simulink model "REL"  (R2022a)
settings: Solver=FixedStepDiscrete  StartTime=0.0  StopTime=10.0  FixedStep=0.01  RelTol=1e-3
libraries: simulink x8, DoorRatSts x4, DoorRlsDriver x2, DoorRlsReq x2
settings Model: Creator=DELL  LastModifiedBy=DELL
settings DataIOCC: SaveFormat=StructureWithTime
settings OptimizationCC: DefaultParameterBehavior=Inlined  EnhancedBackFolding=on  PassReuseOutputArgsAs=Individual arguments  ZeroExternalMemoryAtStartup=off  ZeroInternalMemoryAtStartup=off  OptimizeBlockOrder=speed  DifferentSizesBufferReuse=on  OptimizationCustomize=off  EfficientTunableParamExpr=on
settings DebuggingCC: ParameterTunabilityLossMsg=error
settings ModelReferenceCC: ModelReferenceNumInstancesAllowed=Single
settings SFSimCC: MATLABDynamicMemAlloc=off
settings RTWCC: Description=AUTOSAR  SystemTargetFile=autosar.tlc  GenCodeOnly=on  TemplateMakefile=ert_default_tmf
settings CodeAppCC: ForceParamTrailComments=on  IgnoreCustomStorageClasses=off  OperatorAnnotations=on  SimulinkDataObjDesc=on  SFDataObjDesc=on  InsertBlockDesc=on
settings STFCustomTargetCC: TargetLangStandard=C99 (ISO)  MultiwordLength=256  ParMdlRefBuildCompliant=on  CompOptLevelCompliant=on  IncludeMdlTerminateFcn=off  CombineOutputUpdateFcns=on  SuppressErrorStatus=on  ERTCustomFileBanners=on  SupportNonFinite=off  SupportComplex=off  SupportContinuousTime=off  SupportNonInlinedSFcns=off  RemoveResetFunc=on  MATLABClassNameForMDSCustomization=Simulink.SoftwareTarget.ERTCustomization  AutosarCompliant=on  GRTInterface=off  UseToolchainInfoCompliant=on  LookupTableObjectStructAxisOrder=2,1,3,4,...  LUTObjectStructOrderEvenSpacing=Size,Table,Breakpoints  SystemTargetFile=autosar.tlc
settings ERTTargetCC: TargetLangStandard=C99 (ISO)  ConcurrentExecutionCompliant=off  IncludeMdlTerminateFcn=off  SuppressErrorStatus=on  SupportNonFinite=off  SupportComplex=off  ModelStepFunctionPrototypeControlCompliant=off  CPPClassGenCompliant=off  AutosarCompliant=on  LookupTableObjectStructAxisOrder=2,1,3,4,...  LUTObjectStructOrderEvenSpacing=Size,Table,Breakpoints  InlinedParameterPlacement=NonHierarchical  ERTCustomFileTemplate=example_file_process.tlc

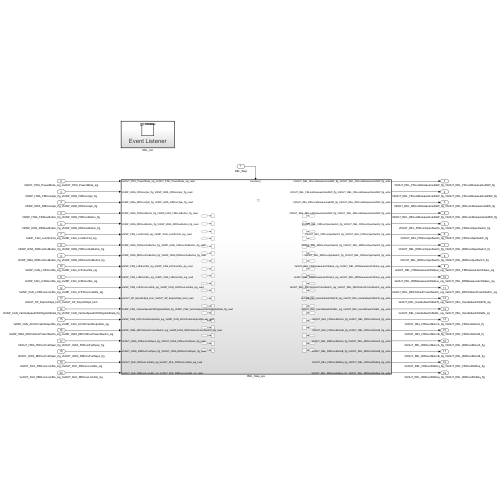
[thumbnail: Simulink's stored preview of the top-level diagram]
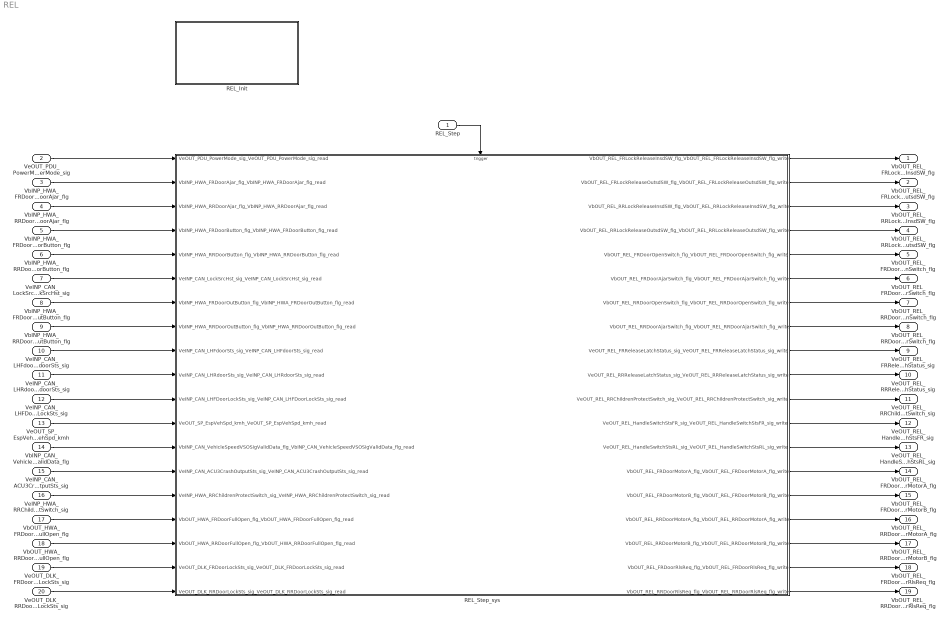
== system REL ==
  REL_Step : Inport  SampleTime=0.01  OutputFunctionCall=on
  VeOUT_PDU_PowerMode_sig_VeOUT_PDU_PowerMode_sig : Inport  Port=2  OutDataTypeStr=UInt8  PortDimensions=1
  VbINP_HWA_FRDoorAjar_flg_VbINP_HWA_FRDoorAjar_flg : Inport  Port=3  OutDataTypeStr=Boolean  PortDimensions=1
  VbINP_HWA_RRDoorAjar_flg_VbINP_HWA_RRDoorAjar_flg : Inport  Port=4  OutDataTypeStr=Boolean  PortDimensions=1
  VbINP_HWA_FRDoorButton_flg_VbINP_HWA_FRDoorButton_flg : Inport  Port=5  OutDataTypeStr=Boolean  PortDimensions=1
  VbINP_HWA_RRDoorButton_flg_VbINP_HWA_RRDoorButton_flg : Inport  Port=6  OutDataTypeStr=Boolean  PortDimensions=1
  VeINP_CAN_LockSrcHst_sig_VeINP_CAN_LockSrcHst_sig : Inport  Port=7  OutDataTypeStr=UInt8  PortDimensions=1
  VbINP_HWA_FRDoorOutButton_flg_VbINP_HWA_FRDoorOutButton_flg : Inport  Port=8  OutDataTypeStr=Boolean  PortDimensions=1
  VbINP_HWA_RRDoorOutButton_flg_VbINP_HWA_RRDoorOutButton_flg : Inport  Port=9  OutDataTypeStr=Boolean  PortDimensions=1
  VeINP_CAN_LHFdoorSts_sig_VeINP_CAN_LHFdoorSts_sig : Inport  Port=10  OutDataTypeStr=UInt8  PortDimensions=1
  VeINP_CAN_LHRdoorSts_sig_VeINP_CAN_LHRdoorSts_sig : Inport  Port=11  OutDataTypeStr=UInt8  PortDimensions=1
  VeINP_CAN_LHFDoorLockSts_sig_VeINP_CAN_LHFDoorLockSts_sig : Inport  Port=12  OutDataTypeStr=UInt8  PortDimensions=1
  VeOUT_SP_EspVehSpd_kmh_VeOUT_SP_EspVehSpd_kmh : Inport  Port=13  OutDataTypeStr=UInt8  PortDimensions=1
  VbINP_CAN_VehicleSpeedVSOSigValidData_flg_VbINP_CAN_VehicleSpeedVSOSigValidData_flg : Inport  Port=14  OutDataTypeStr=Boolean  PortDimensions=1
  VeINP_CAN_ACU3CrashOutputSts_sig_VeINP_CAN_ACU3CrashOutputSts_sig : Inport  Port=15  OutDataTypeStr=UInt8  PortDimensions=1
  VeINP_HWA_RRChildrenProtectSwitch_sig_VeINP_HWA_RRChildrenProtectSwitch_sig : Inport  Port=16  OutDataTypeStr=UInt8  PortDimensions=1
  VbOUT_HWA_FRDoorFullOpen_flg_VbOUT_HWA_FRDoorFullOpen_flg : Inport  Port=17  OutDataTypeStr=Boolean  PortDimensions=1
  VbOUT_HWA_RRDoorFullOpen_flg_VbOUT_HWA_RRDoorFullOpen_flg : Inport  Port=18  OutDataTypeStr=Boolean  PortDimensions=1
  VeOUT_DLK_FRDoorLockSts_sig_VeOUT_DLK_FRDoorLockSts_sig : Inport  Port=19  OutDataTypeStr=UInt8  PortDimensions=1
  VeOUT_DLK_RRDoorLockSts_sig_VeOUT_DLK_RRDoorLockSts_sig : Inport  Port=20  OutDataTypeStr=UInt8  PortDimensions=1
  REL_Init : Subsystem
  REL_Step_sys : Subsystem
  VbOUT_REL_FRLockReleaseInsdSW_flg_VbOUT_REL_FRLockReleaseInsdSW_flg : Outport  OutDataTypeStr=Boolean  PortDimensions=1
  VbOUT_REL_FRLockReleaseOutsdSW_flg_VbOUT_REL_FRLockReleaseOutsdSW_flg : Outport  Port=2  OutDataTypeStr=Boolean  PortDimensions=1
  VbOUT_REL_RRLockReleaseInsdSW_flg_VbOUT_REL_RRLockReleaseInsdSW_flg : Outport  Port=3  OutDataTypeStr=Boolean  PortDimensions=1
  VbOUT_REL_RRLockReleaseOutsdSW_flg_VbOUT_REL_RRLockReleaseOutsdSW_flg : Outport  Port=4  OutDataTypeStr=Boolean  PortDimensions=1
  VbOUT_REL_FRDoorOpenSwitch_flg_VbOUT_REL_FRDoorOpenSwitch_flg : Outport  Port=5  OutDataTypeStr=Boolean  PortDimensions=1
  VbOUT_REL_FRDoorAjarSwitch_flg_VbOUT_REL_FRDoorAjarSwitch_flg : Outport  Port=6  OutDataTypeStr=Boolean  PortDimensions=1
  VbOUT_REL_RRDoorOpenSwitch_flg_VbOUT_REL_RRDoorOpenSwitch_flg : Outport  Port=7  OutDataTypeStr=Boolean  PortDimensions=1
  VbOUT_REL_RRDoorAjarSwitch_flg_VbOUT_REL_RRDoorAjarSwitch_flg : Outport  Port=8  OutDataTypeStr=Boolean  PortDimensions=1
  VeOUT_REL_FRReleaseLatchStatus_sig_VeOUT_REL_FRReleaseLatchStatus_sig : Outport  Port=9  OutDataTypeStr=UInt8  PortDimensions=1
  VeOUT_REL_RRReleaseLatchStatus_sig_VeOUT_REL_RRReleaseLatchStatus_sig : Outport  Port=10  OutDataTypeStr=UInt8  PortDimensions=1
  VeOUT_REL_RRChildrenProtectSwitch_sig_VeOUT_REL_RRChildrenProtectSwitch_sig : Outport  Port=11  OutDataTypeStr=UInt8  PortDimensions=1
  VeOUT_REL_HandleSwitchStsFR_sig_VeOUT_REL_HandleSwitchStsFR_sig : Outport  Port=12  OutDataTypeStr=UInt8  PortDimensions=1
  VeOUT_REL_HandleSwitchStsRL_sig_VeOUT_REL_HandleSwitchStsRL_sig : Outport  Port=13  OutDataTypeStr=UInt8  PortDimensions=1
  VbOUT_REL_FRDoorMotorA_flg_VbOUT_REL_FRDoorMotorA_flg : Outport  Port=14  OutDataTypeStr=Boolean  PortDimensions=1
  VbOUT_REL_FRDoorMotorB_flg_VbOUT_REL_FRDoorMotorB_flg : Outport  Port=15  OutDataTypeStr=Boolean  PortDimensions=1
  VbOUT_REL_RRDoorMotorA_flg_VbOUT_REL_RRDoorMotorA_flg : Outport  Port=16  OutDataTypeStr=Boolean  PortDimensions=1
  VbOUT_REL_RRDoorMotorB_flg_VbOUT_REL_RRDoorMotorB_flg : Outport  Port=17  OutDataTypeStr=Boolean  PortDimensions=1
  VbOUT_REL_FRDoorRlsReq_flg_VbOUT_REL_FRDoorRlsReq_flg : Outport  Port=18  OutDataTypeStr=Boolean  PortDimensions=1
  VbOUT_REL_RRDoorRlsReq_flg_VbOUT_REL_RRDoorRlsReq_flg : Outport  Port=19  OutDataTypeStr=Boolean  PortDimensions=1
  wires:
  VeOUT_PDU_PowerMode_sig_VeOUT_PDU_PowerMode_sig/1 -> REL_Step_sys/1(VeOUT_PDU_PowerMode_sig_VeOUT_PDU_PowerMode_sig_read)
  VbINP_HWA_FRDoorAjar_flg_VbINP_HWA_FRDoorAjar_flg/1 -> REL_Step_sys/2(VbINP_HWA_FRDoorAjar_flg_VbINP_HWA_FRDoorAjar_flg_read)
  VbINP_HWA_RRDoorAjar_flg_VbINP_HWA_RRDoorAjar_flg/1 -> REL_Step_sys/3(VbINP_HWA_RRDoorAjar_flg_VbINP_HWA_RRDoorAjar_flg_read)
  VbINP_HWA_FRDoorButton_flg_VbINP_HWA_FRDoorButton_flg/1 -> REL_Step_sys/4(VbINP_HWA_FRDoorButton_flg_VbINP_HWA_FRDoorButton_flg_read)
  VbINP_HWA_RRDoorButton_flg_VbINP_HWA_RRDoorButton_flg/1 -> REL_Step_sys/5(VbINP_HWA_RRDoorButton_flg_VbINP_HWA_RRDoorButton_flg_read)
  VeINP_CAN_LockSrcHst_sig_VeINP_CAN_LockSrcHst_sig/1 -> REL_Step_sys/6(VeINP_CAN_LockSrcHst_sig_VeINP_CAN_LockSrcHst_sig_read)
  VbINP_HWA_FRDoorOutButton_flg_VbINP_HWA_FRDoorOutButton_flg/1 -> REL_Step_sys/7(VbINP_HWA_FRDoorOutButton_flg_VbINP_HWA_FRDoorOutButton_flg_read)
  VbINP_HWA_RRDoorOutButton_flg_VbINP_HWA_RRDoorOutButton_flg/1 -> REL_Step_sys/8(VbINP_HWA_RRDoorOutButton_flg_VbINP_HWA_RRDoorOutButton_flg_read)
  VeINP_CAN_LHFdoorSts_sig_VeINP_CAN_LHFdoorSts_sig/1 -> REL_Step_sys/9(VeINP_CAN_LHFdoorSts_sig_VeINP_CAN_LHFdoorSts_sig_read)
  VeINP_CAN_LHRdoorSts_sig_VeINP_CAN_LHRdoorSts_sig/1 -> REL_Step_sys/10(VeINP_CAN_LHRdoorSts_sig_VeINP_CAN_LHRdoorSts_sig_read)
  VeINP_CAN_LHFDoorLockSts_sig_VeINP_CAN_LHFDoorLockSts_sig/1 -> REL_Step_sys/11(VeINP_CAN_LHFDoorLockSts_sig_VeINP_CAN_LHFDoorLockSts_sig_read)
  VeOUT_SP_EspVehSpd_kmh_VeOUT_SP_EspVehSpd_kmh/1 -> REL_Step_sys/12(VeOUT_SP_EspVehSpd_kmh_VeOUT_SP_EspVehSpd_kmh_read)
  VbINP_CAN_VehicleSpeedVSOSigValidData_flg_VbINP_CAN_VehicleSpeedVSOSigValidData_flg/1 -> REL_Step_sys/13(VbINP_CAN_VehicleSpeedVSOSigValidData_flg_VbINP_CAN_VehicleSpeedVSOSigValidData_flg_read)
  VeINP_CAN_ACU3CrashOutputSts_sig_VeINP_CAN_ACU3CrashOutputSts_sig/1 -> REL_Step_sys/14(VeINP_CAN_ACU3CrashOutputSts_sig_VeINP_CAN_ACU3CrashOutputSts_sig_read)
  VeINP_HWA_RRChildrenProtectSwitch_sig_VeINP_HWA_RRChildrenProtectSwitch_sig/1 -> REL_Step_sys/15(VeINP_HWA_RRChildrenProtectSwitch_sig_VeINP_HWA_RRChildrenProtectSwitch_sig_read)
  VbOUT_HWA_FRDoorFullOpen_flg_VbOUT_HWA_FRDoorFullOpen_flg/1 -> REL_Step_sys/16(VbOUT_HWA_FRDoorFullOpen_flg_VbOUT_HWA_FRDoorFullOpen_flg_read)
  VbOUT_HWA_RRDoorFullOpen_flg_VbOUT_HWA_RRDoorFullOpen_flg/1 -> REL_Step_sys/17(VbOUT_HWA_RRDoorFullOpen_flg_VbOUT_HWA_RRDoorFullOpen_flg_read)
  VeOUT_DLK_FRDoorLockSts_sig_VeOUT_DLK_FRDoorLockSts_sig/1 -> REL_Step_sys/18(VeOUT_DLK_FRDoorLockSts_sig_VeOUT_DLK_FRDoorLockSts_sig_read)
  VeOUT_DLK_RRDoorLockSts_sig_VeOUT_DLK_RRDoorLockSts_sig/1 -> REL_Step_sys/19(VeOUT_DLK_RRDoorLockSts_sig_VeOUT_DLK_RRDoorLockSts_sig_read)
  REL_Step_sys/1(VbOUT_REL_FRLockReleaseInsdSW_flg_VbOUT_REL_FRLockReleaseInsdSW_flg_write) -> VbOUT_REL_FRLockReleaseInsdSW_flg_VbOUT_REL_FRLockReleaseInsdSW_flg/1
  REL_Step_sys/2(VbOUT_REL_FRLockReleaseOutsdSW_flg_VbOUT_REL_FRLockReleaseOutsdSW_flg_write) -> VbOUT_REL_FRLockReleaseOutsdSW_flg_VbOUT_REL_FRLockReleaseOutsdSW_flg/1
  REL_Step_sys/3(VbOUT_REL_RRLockReleaseInsdSW_flg_VbOUT_REL_RRLockReleaseInsdSW_flg_write) -> VbOUT_REL_RRLockReleaseInsdSW_flg_VbOUT_REL_RRLockReleaseInsdSW_flg/1
  REL_Step_sys/4(VbOUT_REL_RRLockReleaseOutsdSW_flg_VbOUT_REL_RRLockReleaseOutsdSW_flg_write) -> VbOUT_REL_RRLockReleaseOutsdSW_flg_VbOUT_REL_RRLockReleaseOutsdSW_flg/1
  REL_Step_sys/5(VbOUT_REL_FRDoorOpenSwitch_flg_VbOUT_REL_FRDoorOpenSwitch_flg_write) -> VbOUT_REL_FRDoorOpenSwitch_flg_VbOUT_REL_FRDoorOpenSwitch_flg/1
  REL_Step_sys/6(VbOUT_REL_FRDoorAjarSwitch_flg_VbOUT_REL_FRDoorAjarSwitch_flg_write) -> VbOUT_REL_FRDoorAjarSwitch_flg_VbOUT_REL_FRDoorAjarSwitch_flg/1
  REL_Step_sys/7(VbOUT_REL_RRDoorOpenSwitch_flg_VbOUT_REL_RRDoorOpenSwitch_flg_write) -> VbOUT_REL_RRDoorOpenSwitch_flg_VbOUT_REL_RRDoorOpenSwitch_flg/1
  REL_Step_sys/8(VbOUT_REL_RRDoorAjarSwitch_flg_VbOUT_REL_RRDoorAjarSwitch_flg_write) -> VbOUT_REL_RRDoorAjarSwitch_flg_VbOUT_REL_RRDoorAjarSwitch_flg/1
  REL_Step_sys/9(VeOUT_REL_FRReleaseLatchStatus_sig_VeOUT_REL_FRReleaseLatchStatus_sig_write) -> VeOUT_REL_FRReleaseLatchStatus_sig_VeOUT_REL_FRReleaseLatchStatus_sig/1
  REL_Step_sys/10(VeOUT_REL_RRReleaseLatchStatus_sig_VeOUT_REL_RRReleaseLatchStatus_sig_write) -> VeOUT_REL_RRReleaseLatchStatus_sig_VeOUT_REL_RRReleaseLatchStatus_sig/1
  REL_Step_sys/11(VeOUT_REL_RRChildrenProtectSwitch_sig_VeOUT_REL_RRChildrenProtectSwitch_sig_write) -> VeOUT_REL_RRChildrenProtectSwitch_sig_VeOUT_REL_RRChildrenProtectSwitch_sig/1
  REL_Step_sys/12(VeOUT_REL_HandleSwitchStsFR_sig_VeOUT_REL_HandleSwitchStsFR_sig_write) -> VeOUT_REL_HandleSwitchStsFR_sig_VeOUT_REL_HandleSwitchStsFR_sig/1
  REL_Step_sys/13(VeOUT_REL_HandleSwitchStsRL_sig_VeOUT_REL_HandleSwitchStsRL_sig_write) -> VeOUT_REL_HandleSwitchStsRL_sig_VeOUT_REL_HandleSwitchStsRL_sig/1
  REL_Step_sys/14(VbOUT_REL_FRDoorMotorA_flg_VbOUT_REL_FRDoorMotorA_flg_write) -> VbOUT_REL_FRDoorMotorA_flg_VbOUT_REL_FRDoorMotorA_flg/1
  REL_Step_sys/15(VbOUT_REL_FRDoorMotorB_flg_VbOUT_REL_FRDoorMotorB_flg_write) -> VbOUT_REL_FRDoorMotorB_flg_VbOUT_REL_FRDoorMotorB_flg/1
  REL_Step_sys/16(VbOUT_REL_RRDoorMotorA_flg_VbOUT_REL_RRDoorMotorA_flg_write) -> VbOUT_REL_RRDoorMotorA_flg_VbOUT_REL_RRDoorMotorA_flg/1
  REL_Step_sys/17(VbOUT_REL_RRDoorMotorB_flg_VbOUT_REL_RRDoorMotorB_flg_write) -> VbOUT_REL_RRDoorMotorB_flg_VbOUT_REL_RRDoorMotorB_flg/1
  REL_Step_sys/18(VbOUT_REL_FRDoorRlsReq_flg_VbOUT_REL_FRDoorRlsReq_flg_write) -> VbOUT_REL_FRDoorRlsReq_flg_VbOUT_REL_FRDoorRlsReq_flg/1
  REL_Step_sys/19(VbOUT_REL_RRDoorRlsReq_flg_VbOUT_REL_RRDoorRlsReq_flg_write) -> VbOUT_REL_RRDoorRlsReq_flg_VbOUT_REL_RRDoorRlsReq_flg/1
  REL_Step/1 -> REL_Step_sys/Trigger

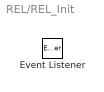
== system REL/REL_Init ==
  Event Listener : EventListener  EventName=reset

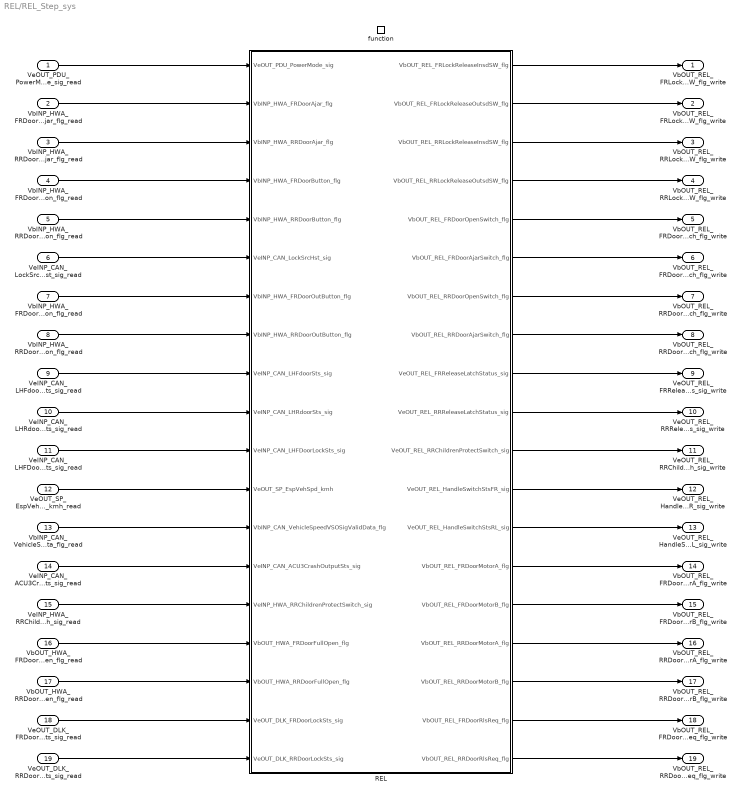
== system REL/REL_Step_sys ==
  VeOUT_PDU_PowerMode_sig_VeOUT_PDU_PowerMode_sig_read : Inport
  VbINP_HWA_FRDoorAjar_flg_VbINP_HWA_FRDoorAjar_flg_read : Inport  Port=2
  VbINP_HWA_RRDoorAjar_flg_VbINP_HWA_RRDoorAjar_flg_read : Inport  Port=3
  VbINP_HWA_FRDoorButton_flg_VbINP_HWA_FRDoorButton_flg_read : Inport  Port=4
  VbINP_HWA_RRDoorButton_flg_VbINP_HWA_RRDoorButton_flg_read : Inport  Port=5
  VeINP_CAN_LockSrcHst_sig_VeINP_CAN_LockSrcHst_sig_read : Inport  Port=6
  VbINP_HWA_FRDoorOutButton_flg_VbINP_HWA_FRDoorOutButton_flg_read : Inport  Port=7
  VbINP_HWA_RRDoorOutButton_flg_VbINP_HWA_RRDoorOutButton_flg_read : Inport  Port=8
  VeINP_CAN_LHFdoorSts_sig_VeINP_CAN_LHFdoorSts_sig_read : Inport  Port=9
  VeINP_CAN_LHRdoorSts_sig_VeINP_CAN_LHRdoorSts_sig_read : Inport  Port=10
  VeINP_CAN_LHFDoorLockSts_sig_VeINP_CAN_LHFDoorLockSts_sig_read : Inport  Port=11
  VeOUT_SP_EspVehSpd_kmh_VeOUT_SP_EspVehSpd_kmh_read : Inport  Port=12
  VbINP_CAN_VehicleSpeedVSOSigValidData_flg_VbINP_CAN_VehicleSpeedVSOSigValidData_flg_read : Inport  Port=13
  VeINP_CAN_ACU3CrashOutputSts_sig_VeINP_CAN_ACU3CrashOutputSts_sig_read : Inport  Port=14
  VeINP_HWA_RRChildrenProtectSwitch_sig_VeINP_HWA_RRChildrenProtectSwitch_sig_read : Inport  Port=15
  VbOUT_HWA_FRDoorFullOpen_flg_VbOUT_HWA_FRDoorFullOpen_flg_read : Inport  Port=16
  VbOUT_HWA_RRDoorFullOpen_flg_VbOUT_HWA_RRDoorFullOpen_flg_read : Inport  Port=17
  VeOUT_DLK_FRDoorLockSts_sig_VeOUT_DLK_FRDoorLockSts_sig_read : Inport  Port=18
  VeOUT_DLK_RRDoorLockSts_sig_VeOUT_DLK_RRDoorLockSts_sig_read : Inport  Port=19
  function : TriggerPort  TriggerType=function-call  VariantControl=(inherit)  SampleTimeType=periodic  SampleTime=-1
  REL : Subsystem
  VbOUT_REL_FRLockReleaseInsdSW_flg_VbOUT_REL_FRLockReleaseInsdSW_flg_write : Outport
      settings: EnsureOutportIsVirtual=on
  VbOUT_REL_FRLockReleaseOutsdSW_flg_VbOUT_REL_FRLockReleaseOutsdSW_flg_write : Outport  Port=2
      settings: EnsureOutportIsVirtual=on
  VbOUT_REL_RRLockReleaseInsdSW_flg_VbOUT_REL_RRLockReleaseInsdSW_flg_write : Outport  Port=3
      settings: EnsureOutportIsVirtual=on
  VbOUT_REL_RRLockReleaseOutsdSW_flg_VbOUT_REL_RRLockReleaseOutsdSW_flg_write : Outport  Port=4
      settings: EnsureOutportIsVirtual=on
  VbOUT_REL_FRDoorOpenSwitch_flg_VbOUT_REL_FRDoorOpenSwitch_flg_write : Outport  Port=5
      settings: EnsureOutportIsVirtual=on
  VbOUT_REL_FRDoorAjarSwitch_flg_VbOUT_REL_FRDoorAjarSwitch_flg_write : Outport  Port=6
      settings: EnsureOutportIsVirtual=on
  VbOUT_REL_RRDoorOpenSwitch_flg_VbOUT_REL_RRDoorOpenSwitch_flg_write : Outport  Port=7
      settings: EnsureOutportIsVirtual=on
  VbOUT_REL_RRDoorAjarSwitch_flg_VbOUT_REL_RRDoorAjarSwitch_flg_write : Outport  Port=8
      settings: EnsureOutportIsVirtual=on
  VeOUT_REL_FRReleaseLatchStatus_sig_VeOUT_REL_FRReleaseLatchStatus_sig_write : Outport  Port=9
      settings: EnsureOutportIsVirtual=on
  VeOUT_REL_RRReleaseLatchStatus_sig_VeOUT_REL_RRReleaseLatchStatus_sig_write : Outport  Port=10
      settings: EnsureOutportIsVirtual=on
  VeOUT_REL_RRChildrenProtectSwitch_sig_VeOUT_REL_RRChildrenProtectSwitch_sig_write : Outport  Port=11
      settings: EnsureOutportIsVirtual=on
  VeOUT_REL_HandleSwitchStsFR_sig_VeOUT_REL_HandleSwitchStsFR_sig_write : Outport  Port=12
      settings: EnsureOutportIsVirtual=on
  VeOUT_REL_HandleSwitchStsRL_sig_VeOUT_REL_HandleSwitchStsRL_sig_write : Outport  Port=13
      settings: EnsureOutportIsVirtual=on
  VbOUT_REL_FRDoorMotorA_flg_VbOUT_REL_FRDoorMotorA_flg_write : Outport  Port=14
      settings: EnsureOutportIsVirtual=on
  VbOUT_REL_FRDoorMotorB_flg_VbOUT_REL_FRDoorMotorB_flg_write : Outport  Port=15
      settings: EnsureOutportIsVirtual=on
  VbOUT_REL_RRDoorMotorA_flg_VbOUT_REL_RRDoorMotorA_flg_write : Outport  Port=16
      settings: EnsureOutportIsVirtual=on
  VbOUT_REL_RRDoorMotorB_flg_VbOUT_REL_RRDoorMotorB_flg_write : Outport  Port=17
      settings: EnsureOutportIsVirtual=on
  VbOUT_REL_FRDoorRlsReq_flg_VbOUT_REL_FRDoorRlsReq_flg_write : Outport  Port=18
      settings: EnsureOutportIsVirtual=on
  VbOUT_REL_RRDoorRlsReq_flg_VbOUT_REL_RRDoorRlsReq_flg_write : Outport  Port=19
      settings: EnsureOutportIsVirtual=on
  wires:
  REL/3(VbOUT_REL_RRLockReleaseInsdSW_flg) -> VbOUT_REL_RRLockReleaseInsdSW_flg_VbOUT_REL_RRLockReleaseInsdSW_flg_write/1
  REL/2(VbOUT_REL_FRLockReleaseOutsdSW_flg) -> VbOUT_REL_FRLockReleaseOutsdSW_flg_VbOUT_REL_FRLockReleaseOutsdSW_flg_write/1
  REL/4(VbOUT_REL_RRLockReleaseOutsdSW_flg) -> VbOUT_REL_RRLockReleaseOutsdSW_flg_VbOUT_REL_RRLockReleaseOutsdSW_flg_write/1
  REL/1(VbOUT_REL_FRLockReleaseInsdSW_flg) -> VbOUT_REL_FRLockReleaseInsdSW_flg_VbOUT_REL_FRLockReleaseInsdSW_flg_write/1
  REL/5(VbOUT_REL_FRDoorOpenSwitch_flg) -> VbOUT_REL_FRDoorOpenSwitch_flg_VbOUT_REL_FRDoorOpenSwitch_flg_write/1
  REL/6(VbOUT_REL_FRDoorAjarSwitch_flg) -> VbOUT_REL_FRDoorAjarSwitch_flg_VbOUT_REL_FRDoorAjarSwitch_flg_write/1
  REL/7(VbOUT_REL_RRDoorOpenSwitch_flg) -> VbOUT_REL_RRDoorOpenSwitch_flg_VbOUT_REL_RRDoorOpenSwitch_flg_write/1
  REL/8(VbOUT_REL_RRDoorAjarSwitch_flg) -> VbOUT_REL_RRDoorAjarSwitch_flg_VbOUT_REL_RRDoorAjarSwitch_flg_write/1
  REL/9(VeOUT_REL_FRReleaseLatchStatus_sig) -> VeOUT_REL_FRReleaseLatchStatus_sig_VeOUT_REL_FRReleaseLatchStatus_sig_write/1
  REL/10(VeOUT_REL_RRReleaseLatchStatus_sig) -> VeOUT_REL_RRReleaseLatchStatus_sig_VeOUT_REL_RRReleaseLatchStatus_sig_write/1
  REL/11(VeOUT_REL_RRChildrenProtectSwitch_sig) -> VeOUT_REL_RRChildrenProtectSwitch_sig_VeOUT_REL_RRChildrenProtectSwitch_sig_write/1
  REL/12(VeOUT_REL_HandleSwitchStsFR_sig) -> VeOUT_REL_HandleSwitchStsFR_sig_VeOUT_REL_HandleSwitchStsFR_sig_write/1
  REL/13(VeOUT_REL_HandleSwitchStsRL_sig) -> VeOUT_REL_HandleSwitchStsRL_sig_VeOUT_REL_HandleSwitchStsRL_sig_write/1
  REL/14(VbOUT_REL_FRDoorMotorA_flg) -> VbOUT_REL_FRDoorMotorA_flg_VbOUT_REL_FRDoorMotorA_flg_write/1
  REL/15(VbOUT_REL_FRDoorMotorB_flg) -> VbOUT_REL_FRDoorMotorB_flg_VbOUT_REL_FRDoorMotorB_flg_write/1
  REL/16(VbOUT_REL_RRDoorMotorA_flg) -> VbOUT_REL_RRDoorMotorA_flg_VbOUT_REL_RRDoorMotorA_flg_write/1
  REL/17(VbOUT_REL_RRDoorMotorB_flg) -> VbOUT_REL_RRDoorMotorB_flg_VbOUT_REL_RRDoorMotorB_flg_write/1
  REL/18(VbOUT_REL_FRDoorRlsReq_flg) -> VbOUT_REL_FRDoorRlsReq_flg_VbOUT_REL_FRDoorRlsReq_flg_write/1
  REL/19(VbOUT_REL_RRDoorRlsReq_flg) -> VbOUT_REL_RRDoorRlsReq_flg_VbOUT_REL_RRDoorRlsReq_flg_write/1
  VbINP_HWA_RRDoorAjar_flg_VbINP_HWA_RRDoorAjar_flg_read/1 -> REL/3(VbINP_HWA_RRDoorAjar_flg)
  VbINP_HWA_FRDoorAjar_flg_VbINP_HWA_FRDoorAjar_flg_read/1 -> REL/2(VbINP_HWA_FRDoorAjar_flg)
  VbINP_HWA_FRDoorButton_flg_VbINP_HWA_FRDoorButton_flg_read/1 -> REL/4(VbINP_HWA_FRDoorButton_flg)
  VeOUT_PDU_PowerMode_sig_VeOUT_PDU_PowerMode_sig_read/1 -> REL/1(VeOUT_PDU_PowerMode_sig)
  VbINP_HWA_RRDoorButton_flg_VbINP_HWA_RRDoorButton_flg_read/1 -> REL/5(VbINP_HWA_RRDoorButton_flg)
  VeINP_CAN_LockSrcHst_sig_VeINP_CAN_LockSrcHst_sig_read/1 -> REL/6(VeINP_CAN_LockSrcHst_sig)
  VbINP_HWA_FRDoorOutButton_flg_VbINP_HWA_FRDoorOutButton_flg_read/1 -> REL/7(VbINP_HWA_FRDoorOutButton_flg)
  VbINP_HWA_RRDoorOutButton_flg_VbINP_HWA_RRDoorOutButton_flg_read/1 -> REL/8(VbINP_HWA_RRDoorOutButton_flg)
  VeINP_CAN_LHFdoorSts_sig_VeINP_CAN_LHFdoorSts_sig_read/1 -> REL/9(VeINP_CAN_LHFdoorSts_sig)
  VeINP_CAN_LHRdoorSts_sig_VeINP_CAN_LHRdoorSts_sig_read/1 -> REL/10(VeINP_CAN_LHRdoorSts_sig)
  VeINP_CAN_LHFDoorLockSts_sig_VeINP_CAN_LHFDoorLockSts_sig_read/1 -> REL/11(VeINP_CAN_LHFDoorLockSts_sig)
  VeOUT_SP_EspVehSpd_kmh_VeOUT_SP_EspVehSpd_kmh_read/1 -> REL/12(VeOUT_SP_EspVehSpd_kmh)
  VbINP_CAN_VehicleSpeedVSOSigValidData_flg_VbINP_CAN_VehicleSpeedVSOSigValidData_flg_read/1 -> REL/13(VbINP_CAN_VehicleSpeedVSOSigValidData_flg)
  VeINP_CAN_ACU3CrashOutputSts_sig_VeINP_CAN_ACU3CrashOutputSts_sig_read/1 -> REL/14(VeINP_CAN_ACU3CrashOutputSts_sig)
  VeINP_HWA_RRChildrenProtectSwitch_sig_VeINP_HWA_RRChildrenProtectSwitch_sig_read/1 -> REL/15(VeINP_HWA_RRChildrenProtectSwitch_sig)
  VbOUT_HWA_FRDoorFullOpen_flg_VbOUT_HWA_FRDoorFullOpen_flg_read/1 -> REL/16(VbOUT_HWA_FRDoorFullOpen_flg)
  VbOUT_HWA_RRDoorFullOpen_flg_VbOUT_HWA_RRDoorFullOpen_flg_read/1 -> REL/17(VbOUT_HWA_RRDoorFullOpen_flg)
  VeOUT_DLK_FRDoorLockSts_sig_VeOUT_DLK_FRDoorLockSts_sig_read/1 -> REL/18(VeOUT_DLK_FRDoorLockSts_sig)
  VeOUT_DLK_RRDoorLockSts_sig_VeOUT_DLK_RRDoorLockSts_sig_read/1 -> REL/19(VeOUT_DLK_RRDoorLockSts_sig)

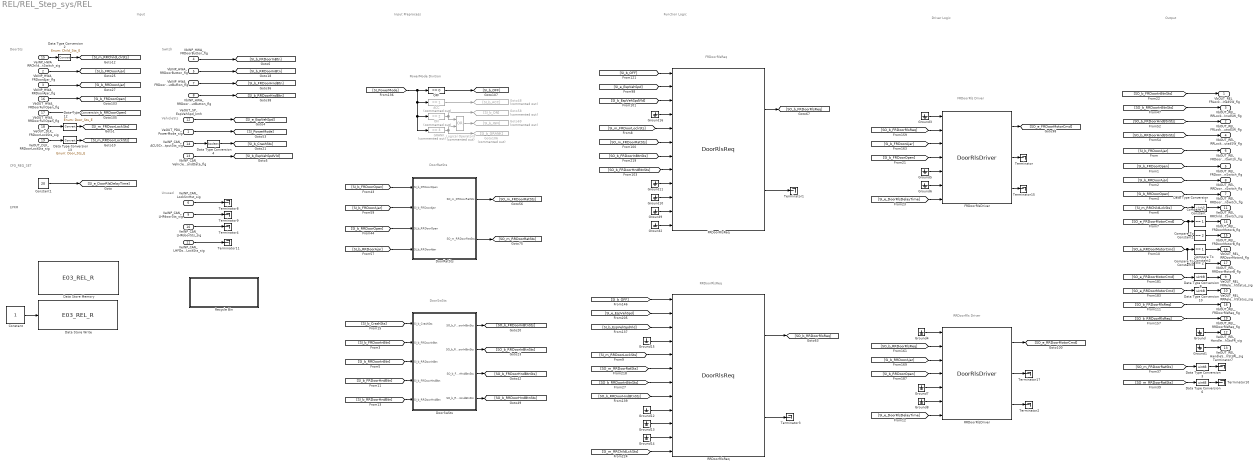
== system REL/REL_Step_sys/REL ==
  note: VehicleSts
  note: Function Logic
  note: Input
  note: Output
  note: Input Preprocess
  note: EPRM
  note: PowerMode Divition
  note: DoorRatSts
  note: Driver Logic
  note: FRDoorRls Driver
  note: FRDoorRlsReq
  note: RRDoorRlsReq
  note: DoorSwSts
  note: Switch
  note: DoorSts
  note: CFG_REQ_SET
  note: Unused
  note: RRDoorRls Driver
  VeOUT_PDU_PowerMode_sig : Inport
  VbINP_HWA_FRDoorAjar_flg : Inport  Port=2
  VbINP_HWA_RRDoorAjar_flg : Inport  Port=3
  VbINP_HWA_FRDoorButton_flg : Inport  Port=4
  VbINP_HWA_RRDoorButton_flg : Inport  Port=5
  VeINP_CAN_LockSrcHst_sig : Inport  Port=6
  VbINP_HWA_FRDoorOutButton_flg : Inport  Port=7
  VbINP_HWA_RRDoorOutButton_flg : Inport  Port=8
  VeINP_CAN_LHFdoorSts_sig : Inport  Port=9
  VeINP_CAN_LHRdoorSts_sig : Inport  Port=10
  VeINP_CAN_LHFDoorLockSts_sig : Inport  Port=11
  VeOUT_SP_EspVehSpd_kmh : Inport  Port=12
  VbINP_CAN_VehicleSpeedVSOSigValidData_flg : Inport  Port=13
  VeINP_CAN_ACU3CrashOutputSts_sig : Inport  Port=14
  VeINP_HWA_RRChildrenProtectSwitch_sig : Inport  Port=15
  VbOUT_HWA_FRDoorFullOpen_flg : Inport  Port=16
  VbOUT_HWA_RRDoorFullOpen_flg : Inport  Port=17
  VeOUT_DLK_FRDoorLockSts_sig : Inport  Port=18
  VeOUT_DLK_RRDoorLockSts_sig : Inport  Port=19
  ACC : simulink/Logic and Bit Operations/Compare To Constant  Commented=on  relop===  const=1  OutDataTypeStr=boolean
  Compare To Constant : simulink/Logic and Bit Operations/Compare To Constant  relop===  const=1  OutDataTypeStr=boolean
  Compare To Constant1 : simulink/Logic and Bit Operations/Compare To Constant  relop===  const=2  OutDataTypeStr=boolean
  Compare To Constant2 : simulink/Logic and Bit Operations/Compare To Constant  relop===  const=1  OutDataTypeStr=boolean
  Compare To Constant3 : simulink/Logic and Bit Operations/Compare To Constant  relop===  const=2  OutDataTypeStr=boolean
  Constant : Constant  OutDataTypeStr=uint8
  Constant1 : Constant  Value=20  OutDataTypeStr=uint8
  Data Store Memory : DataStoreMemory  DataStoreName=E03_REL_R  WriteAfterWriteMsg=warning  ShowAdditionalParam=off  OutDataTypeStr=uint8
  Data Store Write : DataStoreWrite  DataStoreName=E03_REL_R  IndexOptions=Index vector (dialog)  Indices=1  OutputSizes=1
  Data Type Conversion{1,3,6,8,10} (5 alike) : DataTypeConversion  OutDataTypeStr=uint8  SaturateOnIntegerOverflow=off  RndMeth=Floor
  Data Type Conversion12 : DataTypeConversion  OutDataTypeStr=Enum: Door_Sts_E  SaturateOnIntegerOverflow=off  RndMeth=Floor
  Data Type Conversion13 : DataTypeConversion  OutDataTypeStr=Enum: Door_Sts_E  SaturateOnIntegerOverflow=off  RndMeth=Floor
  Data Type Conversion2 : DataTypeConversion  OutDataTypeStr=Enum: Child_Sts_E  SaturateOnIntegerOverflow=off  RndMeth=Floor
  Data Type Conversion4 : DataTypeConversion  OutDataTypeStr=boolean  SaturateOnIntegerOverflow=off  RndMeth=Floor
  DoorRatSts : Stateflow chart  TreatAsAtomicUnit=on
  DoorSwSts : Stateflow chart  TreatAsAtomicUnit=on
  FRDoorRlsDriver : DoorRlsDriver/DoorRlsDriver  SystemSampleTime=-1  VariantActivationTime=update diagram  Latency=0  AutoFrameSizeCalculation=off
  FRDoorRlsReq : DoorRlsReq/DoorRlsReq  SystemSampleTime=-1  VariantActivationTime=update diagram  Latency=0  AutoFrameSizeCalculation=off
  GRANK : simulink/Logic and Bit Operations/Compare To Constant  Commented=on  relop===  const=3  OutDataTypeStr=boolean
  Goto106 : Goto  Commented=on  GotoTag=SI_b_GRANK
  Goto48 : Goto  Commented=on  GotoTag=SI_b_ACC
  Goto58 : Goto  Commented=on  GotoTag=SI_b_ON
  Goto69 : Goto  Commented=on  GotoTag=SI_b_IGN
  Ground{,1..16} (17 alike) : Ground
  Logical Operator3 : Logic  Commented=on  Operator=OR  AllPortsSameDT=off  OutDataTypeStr=boolean
  "OFF " : simulink/Logic and Bit Operations/Compare To Constant  relop===  const=0  OutDataTypeStr=boolean
  ON : simulink/Logic and Bit Operations/Compare To Constant  Commented=on  relop===  const=2  OutDataTypeStr=boolean
  RRDoorRlsDriver : DoorRlsDriver/DoorRlsDriver  SystemSampleTime=-1  VariantActivationTime=update diagram  Latency=0  AutoFrameSizeCalculation=off
  RRDoorRlsReq : DoorRlsReq/DoorRlsReq  SystemSampleTime=-1  VariantActivationTime=update diagram  Latency=0  AutoFrameSizeCalculation=off
  Recycle Bin : Subsystem
  Terminator{,1..4,7..11,15,17} (12 alike) : Terminator
  VbOUT_REL_FRLockReleaseInsdSW_flg : Outport
  VbOUT_REL_FRLockReleaseOutsdSW_flg : Outport  Port=2
  VbOUT_REL_RRLockReleaseInsdSW_flg : Outport  Port=3
  VbOUT_REL_RRLockReleaseOutsdSW_flg : Outport  Port=4
  VbOUT_REL_FRDoorOpenSwitch_flg : Outport  Port=5
  VbOUT_REL_FRDoorAjarSwitch_flg : Outport  Port=6
  VbOUT_REL_RRDoorOpenSwitch_flg : Outport  Port=7
  VbOUT_REL_RRDoorAjarSwitch_flg : Outport  Port=8
  VeOUT_REL_FRReleaseLatchStatus_sig : Outport  Port=9
  VeOUT_REL_RRReleaseLatchStatus_sig : Outport  Port=10
  VeOUT_REL_RRChildrenProtectSwitch_sig : Outport  Port=11
  VeOUT_REL_HandleSwitchStsFR_sig : Outport  Port=12
  VeOUT_REL_HandleSwitchStsRL_sig : Outport  Port=13
  VbOUT_REL_FRDoorMotorA_flg : Outport  Port=14
  VbOUT_REL_FRDoorMotorB_flg : Outport  Port=15
  VbOUT_REL_RRDoorMotorA_flg : Outport  Port=16
  VbOUT_REL_RRDoorMotorB_flg : Outport  Port=17
  VbOUT_REL_FRDoorRlsReq_flg : Outport  Port=18
  VbOUT_REL_RRDoorRlsReq_flg : Outport  Port=19
  wires:
  "OFF "/1 -> [SI_b_OFF]
  [SI_PowerMode] -> "OFF "/1, GRANK/1, ON/1, ACC/1
  ON/1 -> Goto58/1, Logical Operator3/1
  GRANK/1 -> Goto106/1, Logical Operator3/2
  Logical Operator3/1 -> Goto69/1
  ACC/1 -> Goto48/1
  FRDoorRlsDriver/2 -> Terminator/1
  RRDoorRlsDriver/3 -> Terminator2/1
  FRDoorRlsReq/1 -> [SO_b_FRDoorRlsReq]
  RRDoorRlsReq/1 -> [SO_b_RRDoorRlsReq]
  FRDoorRlsDriver/3 -> Terminator15/1
  RRDoorRlsDriver/2 -> Terminator17/1
  [SI_b_OFF] -> FRDoorRlsReq/1
  [SI_e_EspVehSpd] -> FRDoorRlsReq/2
  [SI_b_EspVehSpdVld] -> FRDoorRlsReq/3
  Ground16/1 -> FRDoorRlsReq/4
  [SI_m_FRDoorLockSts] -> FRDoorRlsReq/5
  [SO_m_FRDoorRatSts] -> FRDoorRlsReq/6
  [SO_b_FRDoorInBtnSts] -> FRDoorRlsReq/7
  [SI_b_OFF] -> RRDoorRlsReq/1
  [SI_e_EspVehSpd] -> RRDoorRlsReq/2
  [SI_b_EspVehSpdVld] -> RRDoorRlsReq/3
  Ground15/1 -> RRDoorRlsReq/4
  [SI_m_RRDoorLockSts] -> RRDoorRlsReq/5
  [SO_m_RRDoorRatSts] -> RRDoorRlsReq/6
  [SO_b_RRDoorInBtnSts] -> RRDoorRlsReq/7
  DoorSwSts/1(SO_b_FRDoorInBtnSts) -> [SO_b_FRDoorInBtnSts]
  [SI_b_FRDoorInBtn] -> DoorSwSts/2(SI_b_FRDoorInBtn)
  [SI_b_CrashSts] -> DoorSwSts/1(SI_b_CrashSts)
  [SI_b_RRDoorInBtn] -> DoorSwSts/3(SI_b_RRDoorInBtn)
  [SI_b_FRDoorHndBtn] -> DoorSwSts/4(SI_b_FRDoorHndBtn)
  [SI_b_RRDoorHndBtn] -> DoorSwSts/5(SI_b_RRDoorHndBtn)
  DoorSwSts/2(SO_b_RRDoorInBtnSts) -> [SO_b_RRDoorInBtnSts]
  DoorSwSts/3(SO_b_FRDoorHndBtnSts) -> [SO_b_FRDoorHndBtnSts]
  DoorSwSts/4(SO_b_RRDoorHndBtnSts) -> [SO_b_RRDoorHndBtnSts]
  Constant/1 -> Data Store Write/1
  RRDoorRlsReq/2 -> Terminator3/1
  [SO_m_FRDoorRatSts] -> Data Type Conversion3/1
  [SO_m_RRDoorRatSts] -> Data Type Conversion6/1
  DoorRatSts/1(SO_m_FRDoorRatSts) -> [SO_m_FRDoorRatSts]
  DoorRatSts/2(SO_m_RRDoorRatSts) -> [SO_m_RRDoorRatSts]
  [SO_e_FRDoorMotorCmd] -> Data Type Conversion8/1
  [SO_e_RRDoorMotorCmd] -> Data Type Conversion10/1
  Data Type Conversion12/1 -> [SI_m_FRDoorLockSts]
  Data Type Conversion13/1 -> [SI_m_RRDoorLockSts]
  [SI_b_FRDoorOpen] -> DoorRatSts/1(SI_b_FRDoorOpen)
  [SI_b_RRDoorOpen] -> DoorRatSts/3(SI_b_RRDoorOpen)
  [SI_b_FRDoorAjar] -> DoorRatSts/2(SI_b_FRDoorAjar)
  [SI_b_RRDoorAjar] -> DoorRatSts/4(SI_b_RRDoorAjar)
  VbINP_HWA_FRDoorAjar_flg/1 -> [SI_b_FRDoorAjar]
  VbINP_HWA_RRDoorAjar_flg/1 -> [SI_b_RRDoorAjar]
  VbOUT_HWA_FRDoorFullOpen_flg/1 -> [SI_b_FRDoorOpen]
  VbOUT_HWA_RRDoorFullOpen_flg/1 -> [SI_b_RRDoorOpen]
  VeOUT_DLK_FRDoorLockSts_sig/1 -> Data Type Conversion12/1
  VeOUT_DLK_RRDoorLockSts_sig/1 -> Data Type Conversion13/1
  VeOUT_PDU_PowerMode_sig/1 -> [SI_PowerMode]
  VbINP_HWA_FRDoorButton_flg/1 -> [SI_b_FRDoorInBtn]
  VbINP_HWA_RRDoorButton_flg/1 -> [SI_b_RRDoorInBtn]
  VbINP_HWA_FRDoorOutButton_flg/1 -> [SI_b_FRDoorHndBtn]
  VbINP_HWA_RRDoorOutButton_flg/1 -> [SI_b_RRDoorHndBtn]
  VeINP_CAN_LockSrcHst_sig/1 -> Terminator8/1
  VeINP_CAN_LHFdoorSts_sig/1 -> Terminator9/1
  VeINP_CAN_LHRdoorSts_sig/1 -> Terminator4/1
  VeOUT_SP_EspVehSpd_kmh/1 -> [SI_e_EspVehSpd]
  VbINP_CAN_VehicleSpeedVSOSigValidData_flg/1 -> [SI_b_EspVehSpdVld]
  [SO_b_FRDoorRlsReq] -> VbOUT_REL_FRDoorRlsReq_flg/1
  [SO_b_RRDoorRlsReq] -> VbOUT_REL_RRDoorRlsReq_flg/1
  [SO_b_FRDoorInBtnSts] -> VbOUT_REL_FRLockReleaseInsdSW_flg/1
  [SO_b_FRDoorHndBtnSts] -> VbOUT_REL_FRLockReleaseOutsdSW_flg/1
  [SI_b_FRDoorAjar] -> VbOUT_REL_FRDoorAjarSwitch_flg/1
  Data Type Conversion8/1 -> VeOUT_REL_FRReleaseLatchStatus_sig/1
  [SO_b_RRDoorInBtnSts] -> VbOUT_REL_RRLockReleaseInsdSW_flg/1
  [SO_b_RRDoorHndBtnSts] -> VbOUT_REL_RRLockReleaseOutsdSW_flg/1
  [SI_b_RRDoorOpen] -> VbOUT_REL_RRDoorOpenSwitch_flg/1
  [SI_b_RRDoorAjar] -> VbOUT_REL_RRDoorAjarSwitch_flg/1
  Data Type Conversion10/1 -> VeOUT_REL_RRReleaseLatchStatus_sig/1
  Ground/1 -> VeOUT_REL_HandleSwitchStsFR_sig/1
  Ground1/1 -> VeOUT_REL_HandleSwitchStsRL_sig/1
  Data Type Conversion3/1 -> Terminator7/1
  Data Type Conversion6/1 -> Terminator10/1
  [SO_b_FRDoorHndBtnSts] -> FRDoorRlsReq/8
  Ground11/1 -> FRDoorRlsReq/9
  Ground10/1 -> FRDoorRlsReq/10
  Ground9/1 -> FRDoorRlsReq/11
  Ground2/1 -> FRDoorRlsReq/12
  [SO_b_RRDoorHndBtnSts] -> RRDoorRlsReq/8
  Ground12/1 -> RRDoorRlsReq/9
  Ground13/1 -> RRDoorRlsReq/10
  Ground14/1 -> RRDoorRlsReq/11
  [SI_m_RRChildLckSts] -> RRDoorRlsReq/12
  [SI_m_RRChildLckSts] -> Data Type Conversion1/1
  Data Type Conversion1/1 -> VeOUT_REL_RRChildrenProtectSwitch_sig/1
  Data Type Conversion2/1 -> [SI_m_RRChildLckSts]
  VeINP_HWA_RRChildrenProtectSwitch_sig/1 -> Data Type Conversion2/1
  VeINP_CAN_LHFDoorLockSts_sig/1 -> Terminator11/1
  [SI_b_FRDoorOpen] -> VbOUT_REL_FRDoorOpenSwitch_flg/1
  VeINP_CAN_ACU3CrashOutputSts_sig/1 -> Data Type Conversion4/1
  Data Type Conversion4/1 -> [SI_b_CrashSts]
  FRDoorRlsDriver/1 -> [SO_e_FRDoorMotorCmd]
  Ground3/1 -> FRDoorRlsDriver/1
  [SI_b_FRDoorAjar] -> FRDoorRlsDriver/3
  [SI_b_FRDoorOpen] -> FRDoorRlsDriver/4
  [SO_b_FRDoorRlsReq] -> FRDoorRlsDriver/2
  [SI_e_DoorRlsDelayTime] -> FRDoorRlsDriver/7
  RRDoorRlsDriver/1 -> [SO_e_RRDoorMotorCmd]
  Ground4/1 -> RRDoorRlsDriver/1
  [SI_b_RRDoorOpen] -> RRDoorRlsDriver/4
  [SI_b_RRDoorAjar] -> RRDoorRlsDriver/3
  [SO_b_RRDoorRlsReq] -> RRDoorRlsDriver/2
  [SI_e_DoorRlsDelayTime] -> RRDoorRlsDriver/7
  Ground5/1 -> FRDoorRlsDriver/5
  Ground6/1 -> FRDoorRlsDriver/6
  Ground7/1 -> RRDoorRlsDriver/5
  Ground8/1 -> RRDoorRlsDriver/6
  [SO_e_FRDoorMotorCmd] -> Compare To Constant1/1, Compare To Constant/1
  Compare To Constant/1 -> VbOUT_REL_FRDoorMotorA_flg/1
  Compare To Constant1/1 -> VbOUT_REL_FRDoorMotorB_flg/1
  [SO_e_RRDoorMotorCmd] -> Compare To Constant3/1, Compare To Constant2/1
  Compare To Constant2/1 -> VbOUT_REL_RRDoorMotorA_flg/1
  Compare To Constant3/1 -> VbOUT_REL_RRDoorMotorB_flg/1
  FRDoorRlsReq/2 -> Terminator1/1
  Constant1/1 -> [SI_e_DoorRlsDelayTime]

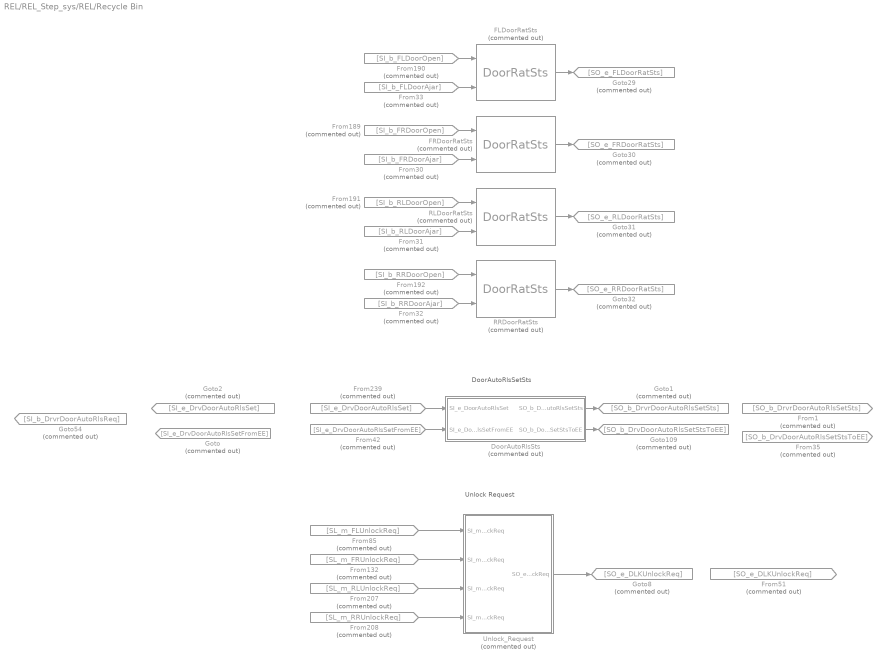
== system REL/REL_Step_sys/REL/Recycle Bin ==
  note: DoorAutoRlsSetSts
  note: Unlock Request
  DoorAutoRlsSts : Stateflow chart  Commented=on  TreatAsAtomicUnit=on
  FLDoorRatSts : DoorRatSts/DoorRatSts  Commented=on  SystemSampleTime=-1  VariantActivationTime=update diagram  Latency=0  AutoFrameSizeCalculation=off
  FRDoorRatSts : DoorRatSts/DoorRatSts  Commented=on  SystemSampleTime=-1  VariantActivationTime=update diagram  Latency=0  AutoFrameSizeCalculation=off
  From1 : From  Commented=on  GotoTag=SO_b_DrvrDoorAutoRlsSetSts
  From132 : From  Commented=on  GotoTag=SL_m_FRUnlockReq
  From189 : From  Commented=on  GotoTag=SI_b_FRDoorOpen
  From190 : From  Commented=on  GotoTag=SI_b_FLDoorOpen
  From191 : From  Commented=on  GotoTag=SI_b_RLDoorOpen
  From192 : From  Commented=on  GotoTag=SI_b_RRDoorOpen
  From207 : From  Commented=on  GotoTag=SL_m_RLUnlockReq
  From208 : From  Commented=on  GotoTag=SL_m_RRUnlockReq
  From239 : From  Commented=on  GotoTag=SI_e_DrvDoorAutoRlsSet
  From30 : From  Commented=on  GotoTag=SI_b_FRDoorAjar
  From31 : From  Commented=on  GotoTag=SI_b_RLDoorAjar
  From32 : From  Commented=on  GotoTag=SI_b_RRDoorAjar
  From33 : From  Commented=on  GotoTag=SI_b_FLDoorAjar
  From35 : From  Commented=on  GotoTag=SO_b_DrvDoorAutoRlsSetStsToEE
  From42 : From  Commented=on  GotoTag=SI_e_DrvDoorAutoRlsSetFromEE
  From51 : From  Commented=on  GotoTag=SO_e_DLKUnlockReq
  From85 : From  Commented=on  GotoTag=SL_m_FLUnlockReq
  Goto : Goto  Commented=on  GotoTag=SI_e_DrvDoorAutoRlsSetFromEE
  Goto1 : Goto  Commented=on  GotoTag=SO_b_DrvrDoorAutoRlsSetSts
  Goto109 : Goto  Commented=on  GotoTag=SO_b_DrvDoorAutoRlsSetStsToEE
  Goto2 : Goto  Commented=on  GotoTag=SI_e_DrvDoorAutoRlsSet
  Goto29 : Goto  Commented=on  GotoTag=SO_e_FLDoorRatSts
  Goto30 : Goto  Commented=on  GotoTag=SO_e_FRDoorRatSts
  Goto31 : Goto  Commented=on  GotoTag=SO_e_RLDoorRatSts
  Goto32 : Goto  Commented=on  GotoTag=SO_e_RRDoorRatSts
  Goto54 : Goto  Commented=on  GotoTag=SI_b_DrvrDoorAutoRlsReq
  Goto8 : Goto  Commented=on  GotoTag=SO_e_DLKUnlockReq
  RLDoorRatSts : DoorRatSts/DoorRatSts  Commented=on  SystemSampleTime=-1  VariantActivationTime=update diagram  Latency=0  AutoFrameSizeCalculation=off
  RRDoorRatSts : DoorRatSts/DoorRatSts  Commented=on  SystemSampleTime=-1  VariantActivationTime=update diagram  Latency=0  AutoFrameSizeCalculation=off
  Unlock_Request : Stateflow chart  Commented=on  TreatAsAtomicUnit=on
  wires:
  FLDoorRatSts/1 -> Goto29/1
  From191/1 -> RLDoorRatSts/1
  FRDoorRatSts/1 -> Goto30/1
  From190/1 -> FLDoorRatSts/1
  From192/1 -> RRDoorRatSts/1
  From189/1 -> FRDoorRatSts/1
  RRDoorRatSts/1 -> Goto32/1
  RLDoorRatSts/1 -> Goto31/1
  From30/1 -> FRDoorRatSts/2
  From32/1 -> RRDoorRatSts/2
  From31/1 -> RLDoorRatSts/2
  From33/1 -> FLDoorRatSts/2
  DoorAutoRlsSts/1(SO_b_DoorAutoRlsSetSts) -> Goto1/1
  DoorAutoRlsSts/2(SO_b_DoorAutoRlsSetStsToEE) -> Goto109/1
  From42/1 -> DoorAutoRlsSts/2(SI_e_DoorAutoRlsSetFromEE)
  From239/1 -> DoorAutoRlsSts/1(SI_e_DoorAutoRlsSet)
  From132/1 -> Unlock_Request/2(SI_m_FRUnlockReq)
  From208/1 -> Unlock_Request/4(SI_m_RRUnlockReq)
  From207/1 -> Unlock_Request/3(SI_m_RLUnlockReq)
  Unlock_Request/1(SO_e_UnlockReq) -> Goto8/1
  From85/1 -> Unlock_Request/1(SI_m_FLUnlockReq)

== stateflow chart REL/REL_Step_sys/REL/Recycle Bin/DoorAutoRlsSts ==
  state DoorLockSet
    (default) -> (junction 127) : /* DoorLockSet */
    DoorLockSet -> (junction 127)
    (junction 127) -> (junction 128) [order 1] : [SI_e_DoorAutoRlsSet == 1 || ...
        | (SI_e_DoorAutoRlsSet != 2 && SL_e_DoorAutoRlsSetBackup == 1)]
    (junction 127) -> (junction 129) [order 2]
    (junction 128) -> (junction 136) : {SO_b_DoorAutoRlsSetSts = 1; ...
        | SO_b_DoorAutoRlsSetStsToEE = 1; ...
        | SL_e_DoorAutoRlsSetBackup = 1}
    (junction 129) -> (junction 130) [order 1] : [SI_e_DoorAutoRlsSet == 2 || ...
        | (SI_e_DoorAutoRlsSet != 1 && SL_e_DoorAutoRlsSetBackup == 2)]
    (junction 129) -> (junction 131) [order 2]
    (junction 130) -> (junction 135) : {SO_b_DoorAutoRlsSetSts = 0; ...
        | SO_b_DoorAutoRlsSetStsToEE = 0; ...
        | SL_e_DoorAutoRlsSetBackup = 2}
    (junction 131) -> (junction 132) [order 1] : [SI_e_DoorAutoRlsSetFromEE == 1]
    (junction 131) -> (junction 151) [order 2]
    (junction 132) -> (junction 134) : {SO_b_DoorAutoRlsSetSts = 1; ...
        | SO_b_DoorAutoRlsSetStsToEE = 1;}
    (junction 151) -> (junction 159) [order 1] : [SI_e_DoorAutoRlsSetFromEE == 0]
    (junction 151) -> (junction 133) [order 2]
    (junction 159) -> (junction 160) : {SO_b_DoorAutoRlsSetSts = 0; ...
        | SO_b_DoorAutoRlsSetStsToEE = 0;}
    (junction 160) -> (junction 133)
    (junction 134) -> (junction 160)
    (junction 135) -> (junction 134)
    (junction 136) -> (junction 135)
    (junction 133) -> (junction 137)
  data: SO_b_DoorAutoRlsSetSts output boolean; SI_e_DoorAutoRlsSet input uint8; SI_e_DoorAutoRlsSetFromEE input uint8; SO_b_DoorAutoRlsSetStsToEE output boolean; SL_e_DoorAutoRlsSetBackup local uint8 =0

== stateflow chart REL/REL_Step_sys/REL/Recycle Bin/Unlock_Request ==
  state req = GetDrvUnlockReq [function]
    (default) -> (junction 216)
    (junction 216) -> (junction 217) [order 1] : [SI_m_FLUnlockReq == Unlock_PE]
    (junction 216) -> (junction 218) [order 2]
    (junction 217) -> (junction 222) : {req = Unlock_PE;}
    (junction 218) -> (junction 219) [order 1] : [SI_m_FLUnlockReq == Unlock_Req]
    (junction 218) -> (junction 220) [order 2] : {req = Unlock_Idle;}
    (junction 219) -> (junction 221) : {req = Unlock_Req;}
    (junction 221) -> (junction 220)
    (junction 222) -> (junction 221)
    (junction 220) -> (junction 223)
  state UnlockReq
    (default) -> (junction 185)
    UnlockReq -> (junction 185)
    (junction 185) -> (junction 186) [order 1] : [(GetDrvUnlockReq() == Unlock_Req && GetPassUnlockReq() == Unlock_Req) || ...
        | GetDrvUnlockReq() == Unlock_PE || ...
        | GetPassUnlockReq() == Unlock_PE]
    (junction 185) -> (junction 187) [order 2]
    (junction 186) -> (junction 194) : {SO_e_UnlockReq = 3;}
    (junction 187) -> (junction 188) [order 1] : [GetDrvUnlockReq() == Unlock_Idle && ...
        | GetPassUnlockReq() == Unlock_Req]
    (junction 187) -> (junction 189) [order 2]
    (junction 188) -> (junction 193) : {SO_e_UnlockReq = 2;}
    (junction 189) -> (junction 190) [order 1] : [GetDrvUnlockReq() == Unlock_Req && ...
        | GetPassUnlockReq() == Unlock_Idle]
    (junction 189) -> (junction 191) [order 2] : {SO_e_UnlockReq = 0;}
    (junction 190) -> (junction 192) : {SO_e_UnlockReq = 1;}
    (junction 192) -> (junction 191)
    (junction 193) -> (junction 192)
    (junction 194) -> (junction 193)
    (junction 191) -> (junction 195)
  state req = GetPassUnlockReq [function]
    (default) -> (junction 232)
    (junction 232) -> (junction 228) [order 1] : [SI_m_FRUnlockReq == Unlock_PE || ...
        | SI_m_RLUnlockReq == Unlock_PE || ...
        | SI_m_RRUnlockReq == Unlock_PE]
    (junction 232) -> (junction 234) [order 2]
    (junction 228) -> (junction 238) : {req = Unlock_PE;}
    (junction 234) -> (junction 237) [order 1] : [SI_m_FRUnlockReq == Unlock_Req || ...
        | SI_m_RLUnlockReq == Unlock_Req || ...
        | SI_m_RRUnlockReq == Unlock_Req]
    (junction 234) -> (junction 240) [order 2] : {req = Unlock_Idle;}
    (junction 237) -> (junction 241) : {req = Unlock_Req;}
    (junction 241) -> (junction 240)
    (junction 238) -> (junction 241)
    (junction 240) -> (junction 239)
  data: req function_output double; req function_output double; SO_e_UnlockReq output uint8; SI_m_FLUnlockReq input Enum: Unlock_Req_E; SI_m_FRUnlockReq input Enum: Unlock_Req_E; SI_m_RLUnlockReq input Enum: Unlock_Req_E; SI_m_RRUnlockReq input Enum: Unlock_Req_E

== stateflow chart REL/REL_Step_sys/REL/DoorRatSts ==
  state DoorRatSts
    (default) -> (junction 42)
    DoorRatSts -> (junction 42)
    (junction 42) -> (junction 53) : {SO_m_FRDoorRatSts = GetDoorRatSts(SI_b_FRDoorAjar, SI_b_FRDoorOpen)}
    (junction 53) -> (junction 45)
    (junction 45) -> (junction 48)
    (junction 48) -> (junction 55)
    (junction 55) -> (junction 57) : {SO_m_RRDoorRatSts = GetDoorRatSts(SI_b_RRDoorAjar, SI_b_RRDoorOpen)}
    (junction 57) -> (junction 58)
    (junction 58) -> (junction 59)
    (junction 59) -> (junction 56)
  state status = GetDoorRatSts(ajar, open) [function]
    (default) -> (junction 24)
    (junction 24) -> (junction 25) [order 1] : [ajar == 0 && open == 0]
    (junction 24) -> (junction 26) [order 2]
    (junction 25) -> (junction 33) : {status = Rat_All_Lock;}
    (junction 26) -> (junction 27) [order 1] : [ajar == 1 && open ==0]
    (junction 26) -> (junction 28) [order 2]
    (junction 27) -> (junction 32) : {status = Rat_Half_Lock;}
    (junction 28) -> (junction 29) [order 1] : [ajar == 1 && open == 1]
    (junction 28) -> (junction 30) [order 2] : {status = Rat_Invalid;}
    (junction 29) -> (junction 31) : {status = Rat_Unlock;}
    (junction 31) -> (junction 30)
    (junction 32) -> (junction 31)
    (junction 33) -> (junction 32)
    (junction 30) -> (junction 34)
  data: ajar function_input double; open function_input double; status function_output double; SI_b_FRDoorOpen input boolean; SO_m_FRDoorRatSts output Enum: Rat_Sts_E; SI_b_FRDoorAjar input boolean; SO_m_RRDoorRatSts output Enum: Rat_Sts_E; SI_b_RRDoorOpen input boolean; SI_b_RRDoorAjar input boolean

== stateflow chart REL/REL_Step_sys/REL/DoorSwSts ==
  state NoCrash
    en,du:
    SO_b_FRDoorInBtnSts = SI_b_FRDoorInBtn;
    SO_b_RRDoorInBtnSts = SI_b_RRDoorInBtn;
    SO_b_FRDoorHndBtnSts = SI_b_FRDoorHndBtn;
    SO_b_RRDoorHndBtnSts = SI_b_RRDoorHndBtn;
  state Crash
    en,du:
    SO_b_FRDoorInBtnSts = 0;
    SO_b_RRDoorInBtnSts = 0;
    SO_b_FRDoorHndBtnSts = 0;
    SO_b_RRDoorHndBtnSts = 0;
  (default) -> NoCrash
  NoCrash -> Crash : [hasChangedTo(SI_b_CrashSts, 1)]
  Crash -> NoCrash : [after(600, tick)]
  data: SO_b_FRDoorInBtnSts output boolean; SI_b_CrashSts input boolean; SI_b_FRDoorInBtn input boolean; SI_b_RRDoorInBtn input boolean; SO_b_RRDoorInBtnSts output boolean; SI_b_FRDoorHndBtn input boolean; SI_b_RRDoorHndBtn input boolean; SO_b_FRDoorHndBtnSts output boolean; SO_b_RRDoorHndBtnSts output boolean
